simulink model "Seesaw_PP"  (R2025b)
settings: Solver=ode4  StartTime=0.0  StopTime=10  FixedStep=0.001  RelTol=1e-3
undefined symbols (not defined in the file): A_sw, B_sw, C_sw, D_sw, Kf, theta0
settings Model: Creator=U448565  LastModifiedBy=U448565

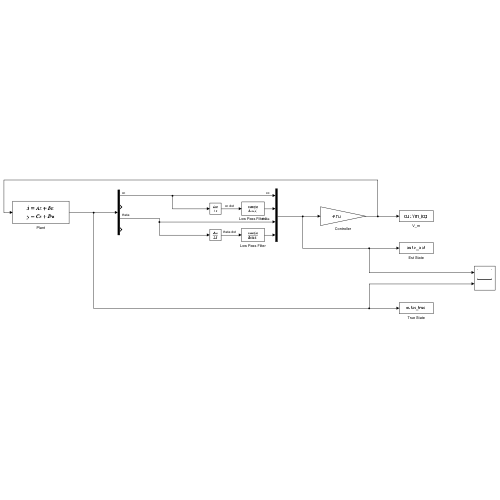
[thumbnail: Simulink's stored preview of the top-level diagram]
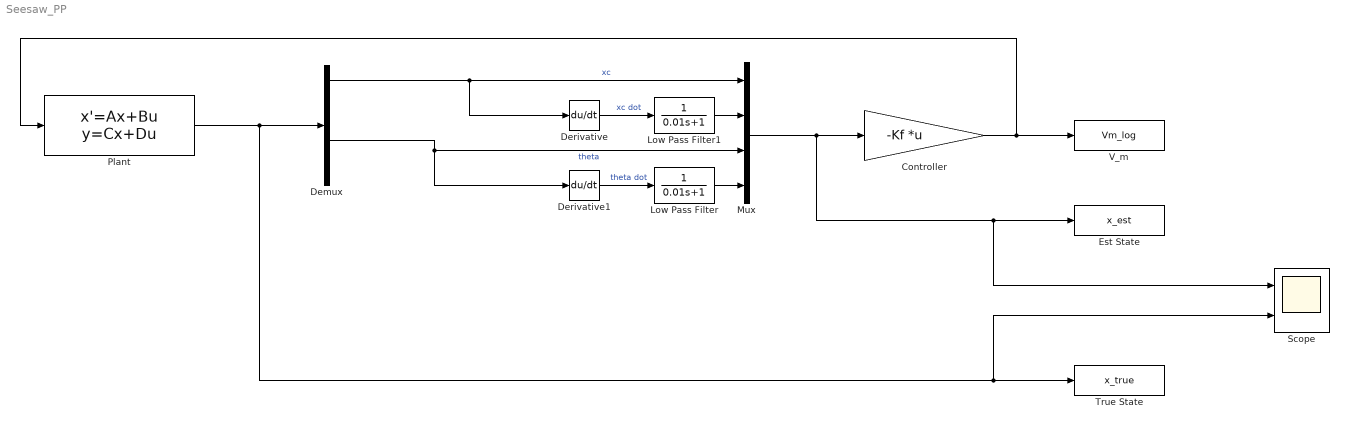
== system Seesaw_PP ==
  Controller : Gain  Gain=-Kf  Multiplication=Matrix(K*u)
  Demux : Demux
  Derivative : Derivative
  Derivative1 : Derivative
  Est State : ToWorkspace  VariableName=x_est  SaveFormat=Timeseries  SampleTime=-1
  Low Pass Filter : TransferFcn  Denominator=[0.01 1]
  Low Pass Filter1 : TransferFcn  Denominator=[0.01 1]
  Mux : Mux
  Plant : StateSpace  A=A_sw  B=B_sw  C=C_sw  D=D_sw  InitialCondition=[0;0;theta0;0]
  Scope : Scope  NumInputPorts=2
      settings: ActiveDisplayYMinimum=-0.20814094676708719  ActiveDisplayYMaximum=0.56753923401338313
  True State : ToWorkspace  VariableName=x_true  SaveFormat=Timeseries  SampleTime=-1
  V_m : ToWorkspace  VariableName=Vm_log  SaveFormat=Timeseries  SampleTime=-1
  wires:
  Plant/1 -> Demux/1, Scope/2, True State/1
  Demux/1 -> Derivative/1, Mux/1  "xc"
  Demux/3 -> Derivative1/1, Mux/3  "theta"
  Controller/1 -> Plant/1, V_m/1
  Derivative/1 -> Low Pass Filter1/1  "xc dot"
  Derivative1/1 -> Low Pass Filter/1  "theta dot"
  Mux/1 -> Controller/1, Scope/1, Est State/1
  Low Pass Filter/1 -> Mux/4
  Low Pass Filter1/1 -> Mux/2
